simulink model "SRR_PDFC"  (R2024b)
settings: Solver=ode4  StartTime=0.0  StopTime=20.0  FixedStep=0.15  RelTol=1e-3
InitFcn:
  | Kp = 1;
  | Kv = 1;
settings Model: Creator=iamma  LastModifiedBy=iamma

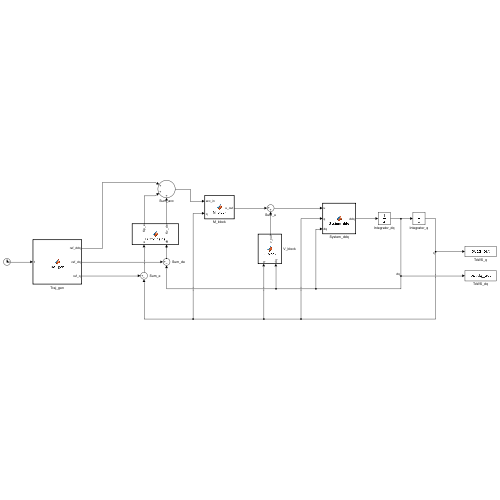
[thumbnail: Simulink's stored preview of the top-level diagram]
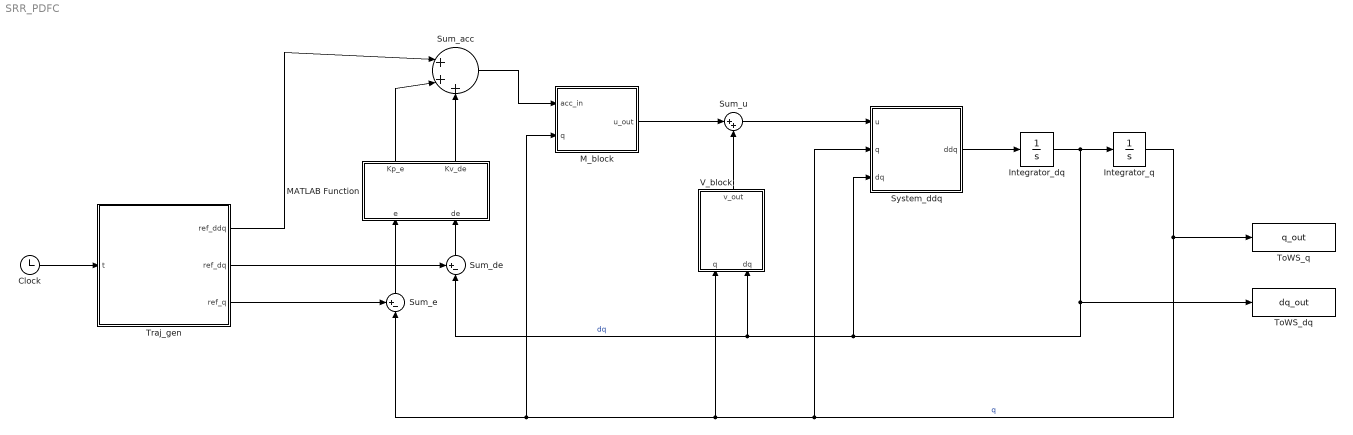
== system SRR_PDFC ==
  Clock : Clock
  Integrator_dq : Integrator  InitialCondition=zeros(4, 1)
  Integrator_q : Integrator  InitialCondition=zeros(4, 1)
  MATLAB Function : MATLAB Function  TreatAsAtomicUnit=on
  M_block : MATLAB Function  TreatAsAtomicUnit=on
  Sum_acc : Sum  Inputs=||+|+|+
  Sum_de : Sum  Inputs=+-|
  Sum_e : Sum  Inputs=+-|
  Sum_u : Sum  Inputs=|++
  System_ddq : MATLAB Function  TreatAsAtomicUnit=on
  ToWS_dq : ToWorkspace  VariableName=dq_out  SampleTime=-1
      settings: Save2DSignal=2-D array (concatenate along first dimension)
  ToWS_q : ToWorkspace  VariableName=q_out  SampleTime=-1
      settings: Save2DSignal=2-D array (concatenate along first dimension)
  Traj_gen : MATLAB Function  TreatAsAtomicUnit=on
  V_block : MATLAB Function  TreatAsAtomicUnit=on
  wires:
  Traj_gen/1(ref_ddq) -> Sum_acc/1
  Traj_gen/2(ref_dq) -> Sum_de/1
  Traj_gen/3(ref_q) -> Sum_e/1
  Sum_acc/1 -> M_block/1(acc_in)
  M_block/1(u_out) -> Sum_u/1
  V_block/1(v_out) -> Sum_u/2
  Sum_u/1 -> System_ddq/1(u)
  System_ddq/1(ddq) -> Integrator_dq/1
  Integrator_dq/1 -> ToWS_dq/1, System_ddq/3(dq), V_block/2(dq), Sum_de/2, Integrator_q/1  "dq"
  Integrator_q/1 -> ToWS_q/1, V_block/1(q), M_block/2(q), Sum_e/2, System_ddq/2(q)  "q"
  Clock/1 -> Traj_gen/1(t)
  Sum_de/1 -> MATLAB Function/2(de)
  Sum_e/1 -> MATLAB Function/1(e)
  MATLAB Function/1(Kp_e) -> Sum_acc/2
  MATLAB Function/2(Kv_de) -> Sum_acc/3

== matlab function SRR_PDFC/M_block ==
  data: acc_in input; u_out output; q input
function u_out = M_block(acc_in, q)
% M(q) * acc_in
p = get_params();
M = calc_M(q, p);
u_out = M * acc_in;
end

== matlab function SRR_PDFC/System_ddq ==
  data: u input; ddq output; q input; dq input
function ddq = System_ddq(u, q, dq)
% ddq = M^{-1} * (u - V)
p = get_params();
M = calc_M(q, p);
V = calc_V(q, dq, p);
ddq = M \ (u - V);
end

== matlab function SRR_PDFC/Traj_gen ==
  data: t input; ref_ddq output; ref_dq output; ref_q output
function [ref_ddq, ref_dq, ref_q] = Traj_gen(t)
[ref_ddq, ref_dq, ref_q] = traj_circular(t);
end

== matlab function SRR_PDFC/MATLAB Function ==
  data: e input; Kp_e output; de input; Kv_de output
function [Kp_e, Kv_de] = Fuzzy_gains(e, de)
% PD-type Fuzzy Controller
% 입력: e (위치 오차 4x1), de (속도 오차 4x1)
% 출력: Kp*e (4x1), Kv*de (4x1)

% x-subsystem만 퍼지 적용 (1번째 성분)
% 나머지는 고정 이득
Kp_base = 1.0;
Kv_base = 1.0;

% x-subsystem 퍼지 이득
Kp_x = fuzzy_gain(e(1), de(1), Kp_base);
Kv_x = fuzzy_gain(de(1), e(1), Kv_base);

Kp_e  = [Kp_x * e(1);  Kp_base * e(2);  Kp_base * e(3);  Kp_base * e(4)];
Kv_de = [Kv_x * de(1); Kv_base * de(2); Kv_base * de(3); Kv_base * de(4)];
end

function K = fuzzy_gain(err, derr, K_base)
% 삼각형 멤버십 함수 기반 퍼지 이득 조정
% 논문 Table II 룰 베이스 구현

% 언어 변수 정의 (NL, NM, NS, ZR, PS, PM, PL)
centers = [-3, -2, -1, 0, 1, 2, 3];
scale_e  = 1.0;
scale_de = 1.0;

% 멤버십 계산
mu_e  = trimf_vector(err  / scale_e,  centers);
mu_de = trimf_vector(derr / scale_de, centers);

% 룰 베이스 (논문 Table II)
rule_base = [
    0, 1, 2, 3, 3, 3, 3;   % PL
    -1, 0, 1, 2, 3, 3, 3;  % PM
    -2,-1, 0, 1, 2, 3, 3;  % PS
    -3,-2,-1, 0, 1, 2, 3;  % ZR
    -3,-3,-2,-1, 0, 1, 2;  % NS
    -3,-3,-3,-2,-1, 0, 1;  % NM
    -3,-3,-3,-3,-2,-1, 0   % NL
];

% 중심법(centroid) defuzzification
numerator   = 0;
denominator = 0;
for i = 1:7
    for j = 1:7
        firing = min(mu_e(i), mu_de(j));
        output_center = rule_base(8-i, j);
        numerator   = numerator   + firing * output_center;
        denominator = denominator + firing;
    end
end

if denominator > 1e-10
    delta_K = numerator / denominator;
else
    delta_K = 0;
end

% 기본 이득에 퍼지 조정값 더하기
K = max(0.1, K_base + 0.5 * delta_K);
end

function mu = trimf_vector(x, centers)
% 삼각형 멤버십 함수 벡터 계산
n  = length(centers);
mu = zeros(1, n);
for i = 1:n
    if i == 1
        mu(i) = trimf(x, centers(1)-1, centers(1), centers(2));
    elseif i == n
        mu(i) = trimf(x, centers(n-1), centers(n), centers(n)+1);
    else
        mu(i) = trimf(x, centers(i-1), centers(i), centers(i+1));
    end
end
end

function y = trimf(x, a, b, c)
% 삼각형 멤버십 함수
if x <= a || x >= c
    y = 0;
elseif x <= b
    y = (x - a) / (b - a);
else
    y = (c - x) / (c - b);
end
end

== matlab function SRR_PDFC/V_block ==
  data: q input; dq input; v_out output
function v_out = V_block(q, dq)
% V(q, dq) 비선형 항
p = get_params();
v_out = calc_V(q, dq, p);
end
